simulink model "helipid"  (Simulink 7.7)
settings: Solver=ode45  StartTime=0.0  StopTime=2  RelTol=1e-3
values from neighbouring files (symbols this model uses):
  m = 97.85/2.20462262    (= 44.3840134417)    [heli_parameter.m]    (also in lin_thrust_countertorque.m; parameter.m)
undefined symbols (not defined in the file or in its folder): s
libraries: simulink x3, aerolib6dofsys x2, aerolibconvert2 x2, aerolibanim x1
settings Model: Creator=Administrator  LastModifiedBy=Li

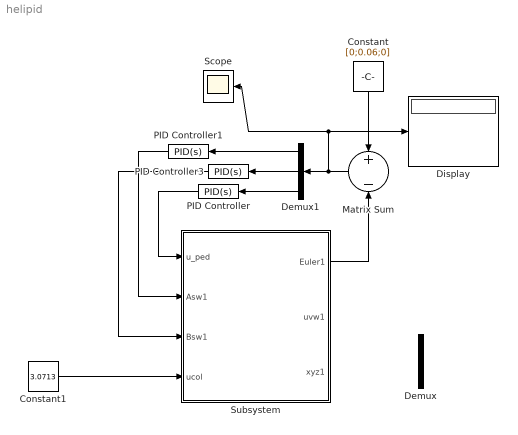
== system helipid ==
  Constant : Constant  Value=[0;0.06;0]
  Constant1 : Constant  Value=3.0713
  Demux : Demux  Outputs=3
  Demux1 : Demux  Outputs=3
  Display : Display
  Matrix Sum : Sum  Inputs=+-
  PID Controller : simulink/Continuous/PID Controller  SystemSampleTime=-1  Controller=PID  TimeDomain=Continuous-time  SampleTime=1  IntegratorMethod=Forward Euler  FilterMethod=Forward Euler  Form=Parallel  P=1  I=1  D=0  N=100  InitialConditionSource=internal  InitialConditionForIntegrator=0  InitialConditionForFilter=0  ExternalReset=none  LimitOutput=off  UpperSaturationLimit=inf  LowerSaturationLimit=-inf  LinearizeAsGain=off  AntiWindupMode=none  Kb=1  TrackingMode=off  Kt=1  PParamMin=[]  PParamMax=[]  IParamMin=[]  IParamMax=[]  DParamMin=[]  DParamMax=[]  NParamMin=[]  NParamMax=[]  KbParamMin=[]  KbParamMax=[]  KtParamMin=[]  KtParamMax=[]  POutMin=[]  POutMax=[]  IOutMin=[]  IOutMax=[]  DOutMin=[]  DOutMax=[]  NOutMin=[]  NOutMax=[]  KbOutMin=[]  KbOutMax=[]  KtOutMin=[]  KtOutMax=[]  IntegratorOutMin=[]  IntegratorOutMax=[]  FilterOutMin=[]  FilterOutMax=[]  SumOutMin=[]  SumOutMax=[]  SumI1OutMin=[]  SumI1OutMax=[]  SumI2OutMin=[]  SumI2OutMax=[]  SumI3OutMin=[]  SumI3OutMax=[]  SumDOutMin=[]  SumDOutMax=[]  SaturationOutMin=[]  SaturationOutMax=[]  IntegratorContinuousStateAttributes=''  IntegratorStateMustResolveToSignalObject=off  IntegratorRTWStateStorageClass=Auto  FilterContinuousStateAttributes=''  FilterStateMustResolveToSignalObject=off  FilterRTWStateStorageClass=Auto
  PID Controller1 : simulink/Continuous/PID Controller  SystemSampleTime=-1  Controller=PID  TimeDomain=Continuous-time  SampleTime=1  IntegratorMethod=Forward Euler  FilterMethod=Forward Euler  Form=Parallel  P=2  I=1  D=0.2  N=100  InitialConditionSource=internal  InitialConditionForIntegrator=0  InitialConditionForFilter=0  ExternalReset=none  LimitOutput=off  UpperSaturationLimit=inf  LowerSaturationLimit=-inf  LinearizeAsGain=off  AntiWindupMode=none  Kb=1  TrackingMode=off  Kt=1  PParamMin=[]  PParamMax=[]  IParamMin=[]  IParamMax=[]  DParamMin=[]  DParamMax=[]  NParamMin=[]  NParamMax=[]  KbParamMin=[]  KbParamMax=[]  KtParamMin=[]  KtParamMax=[]  POutMin=[]  POutMax=[]  IOutMin=[]  IOutMax=[]  DOutMin=[]  DOutMax=[]  NOutMin=[]  NOutMax=[]  KbOutMin=[]  KbOutMax=[]  KtOutMin=[]  KtOutMax=[]  IntegratorOutMin=[]  IntegratorOutMax=[]  FilterOutMin=[]  FilterOutMax=[]  SumOutMin=[]  SumOutMax=[]  SumI1OutMin=[]  SumI1OutMax=[]  SumI2OutMin=[]  SumI2OutMax=[]  SumI3OutMin=[]  SumI3OutMax=[]  SumDOutMin=[]  SumDOutMax=[]  SaturationOutMin=[]  SaturationOutMax=[]  IntegratorContinuousStateAttributes=''  IntegratorStateMustResolveToSignalObject=off  IntegratorRTWStateStorageClass=Auto  FilterContinuousStateAttributes=''  FilterStateMustResolveToSignalObject=off  FilterRTWStateStorageClass=Auto
  PID Controller3 : simulink/Continuous/PID Controller  SystemSampleTime=-1  Controller=PID  TimeDomain=Continuous-time  SampleTime=1  IntegratorMethod=Forward Euler  FilterMethod=Forward Euler  Form=Parallel  P=1.25  I=0.5  D=0.0474823432420019  N=10  InitialConditionSource=internal  InitialConditionForIntegrator=0  InitialConditionForFilter=0  ExternalReset=none  LimitOutput=off  UpperSaturationLimit=inf  LowerSaturationLimit=-inf  LinearizeAsGain=off  AntiWindupMode=none  Kb=1  TrackingMode=off  Kt=1  PParamMin=[]  PParamMax=[]  IParamMin=[]  IParamMax=[]  DParamMin=[]  DParamMax=[]  NParamMin=[]  NParamMax=[]  KbParamMin=[]  KbParamMax=[]  KtParamMin=[]  KtParamMax=[]  POutMin=[]  POutMax=[]  IOutMin=[]  IOutMax=[]  DOutMin=[]  DOutMax=[]  NOutMin=[]  NOutMax=[]  KbOutMin=[]  KbOutMax=[]  KtOutMin=[]  KtOutMax=[]  IntegratorOutMin=[]  IntegratorOutMax=[]  FilterOutMin=[]  FilterOutMax=[]  SumOutMin=[]  SumOutMax=[]  SumI1OutMin=[]  SumI1OutMax=[]  SumI2OutMin=[]  SumI2OutMax=[]  SumI3OutMin=[]  SumI3OutMax=[]  SumDOutMin=[]  SumDOutMax=[]  SaturationOutMin=[]  SaturationOutMax=[]  IntegratorContinuousStateAttributes=''  IntegratorStateMustResolveToSignalObject=off  IntegratorRTWStateStorageClass=Auto  FilterContinuousStateAttributes=''  FilterStateMustResolveToSignalObject=off  FilterRTWStateStorageClass=Auto
  Scope : Scope
      settings: SaveName=ScopeData13
  Subsystem : Subsystem
  wires:
  Constant/1 -> Matrix Sum/1
  Subsystem/1(Euler1) -> Matrix Sum/2
  Matrix Sum/1 -> Demux1/1, Display/1, Scope/1
  Demux1/3 -> PID Controller/1
  PID Controller/1 -> Subsystem/1(u_ped)
  Demux1/1 -> PID Controller1/1
  PID Controller1/1 -> Subsystem/2(Asw1)
  Demux1/2 -> PID Controller3/1
  PID Controller3/1 -> Subsystem/3(Bsw1)
  Constant1/1 -> Subsystem/4(ucol)

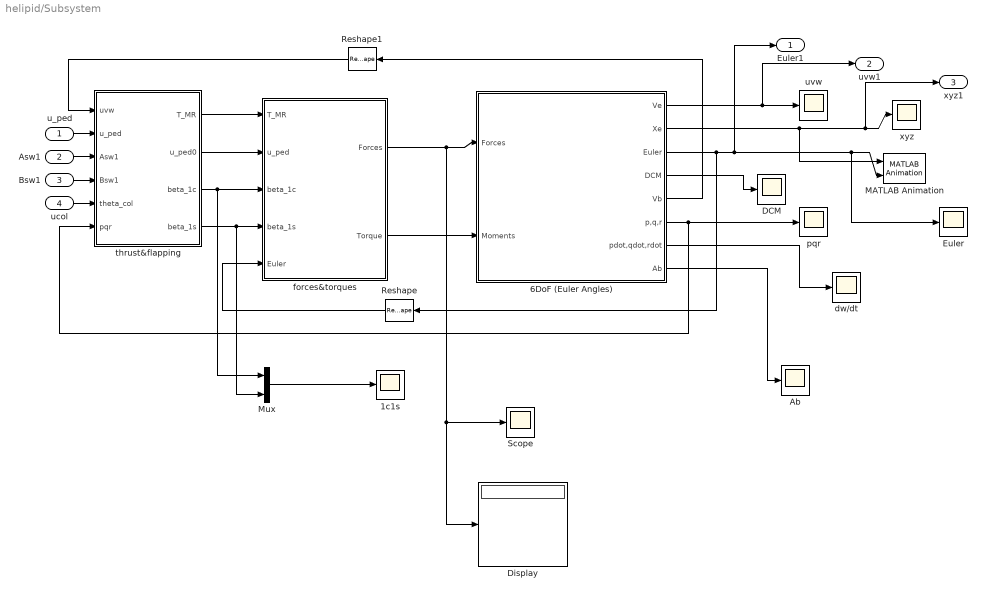
== system helipid/Subsystem ==
  u_ped : Inport
  Asw1 : Inport  Port=2
  Bsw1 : Inport  Port=3
  ucol : Inport  Port=4
  1c1s : Scope
      settings: YMin=1.5e-007  YMax=6.75e-007
  6DoF (Euler Angles) : Subsystem  AncestorBlock=aerolib6dof2/6DoF (Euler Angles)  mask(6DoF EoM (Body Axis)){units=Metric (MKS), mtype=Fixed, rep=Euler Angles, xme_0=[0;0;0], Vm_0=[0;0;0], eul_0=[0;0;0], pm_0=[0;0;0], mass_0=44.38401344172002, mass_e=0.5, mass_f=2.0, inertia=[1.4667965 0 0;0 4.5766695 0;0 0 4.407], inertia_e=eye(3), inertia_f=2*eye(3), k_quat=1.0}
      mask prompts: mtype "Mass type:"; rep "Representation:"; xme_0 "Initial position in inertial axes [Xe,Ye,Ze]:"; Vm_0 "Initial velocity in body axes [U,v,w]:"; eul_0 "Initial Euler orientation [roll, pitch, yaw]:"; pm_0 "Initial body rotation rates [p,q,r]:"; mass_0 "Initial mass:"; mass_e "Empty mass:"; mass_f "Full mass:"; inertia_e "Empty inertia matrix:"; inertia_f "Full inertia matrix:"; k_quat "Gain for quaternion normalization:"
      mask help: Integrate the six-degrees-of-freedom equations of motion in body axis.
      mask init:
      | [x y xp yp highstr lowstr maxy miny]=aeroimage('sixdofbody',gcbh);
      | ports=aeroicon('aeroblk6dofbody','icon');
      mask Help: eval('asbhelp(''sixdof_euler_angles'')');
      mask StyleString: popup(Metric (MKS)|English (Velocity in ft/s)|English (Velocity in kts)),popup(Fixed|Simple Variable|Custom Variable),popup(Euler Angles|Quaternion),edit,edit,edit,edit,edit,edit,edit,edit,edit,edit,edit
      mask CallbackString: |aeroicon('aeroblk6dofbody');|aeroicon('aeroblk6dofbody');|||||||||||
      mask Display:
      | port_label(ports(1).type,ports(1).port,ports(1).txt,'texmode','on');
      | port_label(ports(2).type,ports(2).port,ports(2).txt,'texmode','on');
      | port_label(ports(3).type,ports(3).port,ports(3).txt,'texmode','on');
      | port_label(ports(4).type,ports(4).port,ports(4).txt,'texmode','on');
      | port_label(ports(5).type,ports(5).port,ports(5).txt,'texmode','on');
      | port_label(ports(6).type,ports(6).port,ports(6).txt,'texmode','on');
      | port_label(ports(7).type,ports(7).port,ports(7).txt,'texmode','on');
      | port_label(ports(8).type,ports(8).port,ports(8).txt,'texmode','on');
      | port_label(ports(9).type,ports(9).port,ports(9).txt,'texmode','on');
      | port_label(ports(10).type,ports(10).port,ports(10).txt,'texmode','on');
      | port_label(ports(11).type,ports(11).port,ports(11).txt,'texmode','on');
      | port_label(ports(12).type,ports(12).port,ports(12).txt,'texmode','on');
      | port_label(ports(13).type,ports(13).port,ports(13).txt,'texmode','on');
      | port_label(ports(14).type,ports(14).port,ports(14).txt,'texmode','on');
      | port_label(ports(15).type,ports(15).port,ports(15).txt,'texmode','on');
      | text(0.5,maxy+0.065,highstr{:},'horizontalAlignment','center')
      | text(0.5,miny-0.05,lowstr{:},'horizontalAlignment','center')
      | plot(x,y);
      | patch(xp, yp);
  Ab : Scope
      settings: YMin=-2.5  YMax=0  SaveName=ScopeData12
  DCM : Scope
      settings: YMin=-2.5  YMax=0  SaveName=ScopeData11
  Display : Display
  Euler : Scope
      settings: YMin=-2.5  YMax=0
  MATLAB Animation : aerolibanim/MATLAB Animation  Vehicles=1  Geometries='astredwedge.mat'  BoundingBoxCoordinates=[-50,50,-50,50,-50,50]  CameraOffset=[-150,0,0]  CameraViewAngle=3  SampleTime=0.1  FigurePosition=[697,108,638,514]
  Mux : Mux  Inputs=2
  Reshape : Reshape  OutputDimensionality=Column vector (2-D)
  Reshape1 : Reshape  OutputDimensionality=Column vector (2-D)
  Scope : Scope
      settings: YMin=-2.5  YMax=0  SaveName=ScopeData2
  dw/dt : Scope
      settings: YMin=-2.5  YMax=0  SaveName=ScopeData3
  forces&torques : Subsystem  mask{mass0=44.384, AQ=0.00036, BQ=0.01, lm=0, ym=0, hm=0.2, Lt=1.2, Ht=0}
  pqr : Scope
      settings: YMin=-2.5  YMax=0  SaveName=ScopeData5
  thrust&flapping : Subsystem  mask{Ksw=0.2, Kcr=0.8, T_old=10, vi0=1, theta_twist=4.864e-4, theta_0=0.07}
  uvw : Scope
      settings: YMin=-2.5  YMax=0  SaveName=ScopeData6
  xyz : Scope
      settings: YMin=-2.5  YMax=0  SaveName=ScopeData7
  Euler1 : Outport
  uvw1 : Outport  Port=2
  xyz1 : Outport  Port=3
  wires:
  forces&torques/1(Forces) -> 6DoF (Euler Angles)/1(Forces), Scope/1, Display/1
  6DoF (Euler Angles)/6(p,q,r) -> thrust&flapping/6(pqr), pqr/1
  6DoF (Euler Angles)/3(Euler) -> Reshape/1, MATLAB Animation/2, Euler/1, Euler1/1
  thrust&flapping/1(T_MR) -> forces&torques/1(T_MR)
  thrust&flapping/2(u_ped0) -> forces&torques/2(u_ped)
  Reshape/1 -> forces&torques/5(Euler)
  6DoF (Euler Angles)/5(Vb) -> Reshape1/1
  Reshape1/1 -> thrust&flapping/1(uvw)
  thrust&flapping/3(beta_1c) -> forces&torques/3(beta_1c), Mux/1
  thrust&flapping/4(beta_1s) -> forces&torques/4(beta_1s), Mux/2
  forces&torques/2(Torque) -> 6DoF (Euler Angles)/2(Moments)
  Mux/1 -> 1c1s/1
  6DoF (Euler Angles)/1(Ve) -> uvw/1, uvw1/1
  6DoF (Euler Angles)/2(Xe) -> MATLAB Animation/1, xyz/1, xyz1/1
  6DoF (Euler Angles)/7(pdot,qdot,rdot) -> dw/dt/1
  6DoF (Euler Angles)/4(DCM) -> DCM/1
  u_ped/1 -> thrust&flapping/2(u_ped)
  Asw1/1 -> thrust&flapping/3(Asw1)
  Bsw1/1 -> thrust&flapping/4(Bsw1)
  ucol/1 -> thrust&flapping/5(theta_col)
  6DoF (Euler Angles)/8(Ab) -> Ab/1

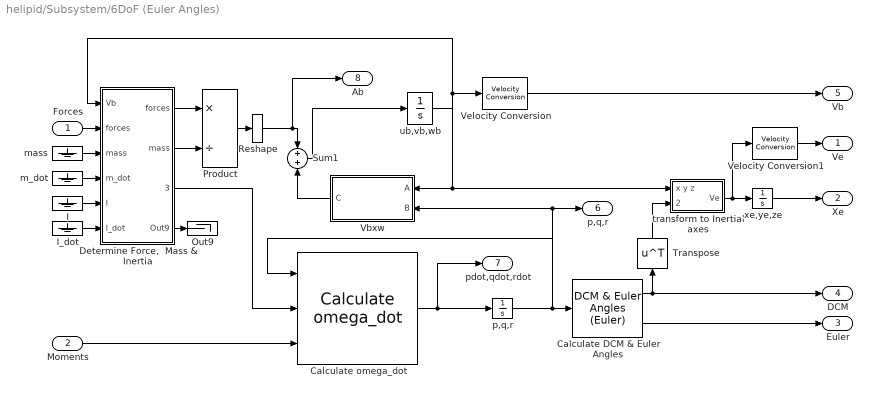
== system helipid/Subsystem/6DoF (Euler Angles) ==
  Forces : Inport
  Moments : Inport  Port=2
  Calculate DCM & Euler Angles : aerolib6dofsys/DCM & Euler Angles (Euler)  SystemSampleTime=-1
  Calculate omega_dot : aerolib6dofsys/Calculate omega_dot  SystemSampleTime=-1
  "Determine Force,  Mass & Inertia" : Subsystem  AncestorBlock=aerolib6dofsys/Mass & Inertia (fixed)
      mask Type: Mass & Inertia (fixed)
  I : Ground
  I_dot : Ground
  Out9 : Terminator
  Product : Product  Inputs=*/  SaturateOnIntegerOverflow=on  OutDataTypeStr=Inherit: Same as first input
  Reshape : Reshape  OutputDimensionality=Column vector (2-D)
  Sum1 : Sum  SaturateOnIntegerOverflow=on  InputSameDT=on  OutDataTypeStr=Inherit: Same as first input
  Transpose : Math  Operator=transpose  SaturateOnIntegerOverflow=on
  Vbxw : Subsystem  AncestorBlock=aerolibutil/3x3 Cross Product  mask(CrossProduct){}
      mask help: Calculate the cross product of two 3-by-1 vectors.
      mask init:
      | aeroicon('aeroblk');
      mask Help: eval('asbhelp(''threebythree_cross_product'')');
      mask Display:
      | text(.5,.5,'Cross\nProduct\nC = AxB', ...
      | 	'HorizontalAlignment','Center',...
      | 	'VerticalAlignment','middle')
  Velocity Conversion : aerolibconvert2/Velocity Conversion  SystemSampleTime=-1  IU=m/s  OU=m/s
  Velocity Conversion1 : aerolibconvert2/Velocity Conversion  SystemSampleTime=-1  IU=m/s  OU=m/s
  m_dot : Ground
  mass : Ground
  "p,q,r " : Integrator  InitialCondition=pm_0
  "transform to Inertial axes " : Subsystem
      mask Type: Vector Transformation
      mask Display: disp('L_EB')
  ub,vb,wb : Integrator  InitialCondition=convvel(Vm_0,'m/s','m/s')
  xe,ye,ze : Integrator  InitialCondition=xme_0
  Ve : Outport
  Xe : Outport  Port=2
  Euler : Outport  Port=3
  DCM : Outport  Port=4
  Vb : Outport  Port=5
  p,q,r : Outport  Port=6
  pdot,qdot,rdot : Outport  Port=7
  Ab : Outport  Port=8
  wires:
  "Determine Force,  Mass & Inertia"/1("forces ") -> Product/1
  I_dot/1 -> "Determine Force,  Mass & Inertia"/6(I_dot)
  I/1 -> "Determine Force,  Mass & Inertia"/5(I)
  Calculate omega_dot/1 -> "p,q,r "/1, pdot,qdot,rdot/1
  "Determine Force,  Mass & Inertia"/4(Out9) -> Out9/1
  m_dot/1 -> "Determine Force,  Mass & Inertia"/4(m_dot)
  "Determine Force,  Mass & Inertia"/2(mass) -> Product/2
  mass/1 -> "Determine Force,  Mass & Inertia"/3("mass ")
  Transpose/1 -> "transform to Inertial axes "/2(transform coefficients)
  Calculate DCM & Euler Angles/1 -> Transpose/1, DCM/1
  Forces/1 -> "Determine Force,  Mass & Inertia"/2(forces)
  Moments/1 -> Calculate omega_dot/3
  "p,q,r "/1 -> Calculate omega_dot/1, Calculate DCM & Euler Angles/1, Vbxw/2(B), p,q,r/1
  "transform to Inertial axes "/1(Ve) -> xe,ye,ze/1, Velocity Conversion1/1
  xe,ye,ze/1 -> Xe/1
  Sum1/1 -> ub,vb,wb/1
  ub,vb,wb/1 -> "Determine Force,  Mass & Inertia"/1(Vb), Vbxw/1(A), "transform to Inertial axes "/1(x y z), Velocity Conversion/1
  Vbxw/1(C) -> Sum1/2
  Calculate DCM & Euler Angles/2 -> Euler/1
  "Determine Force,  Mass & Inertia"/3("inertia, 0") -> Calculate omega_dot/2
  Velocity Conversion/1 -> Vb/1
  Velocity Conversion1/1 -> Ve/1
  Product/1 -> Reshape/1
  Reshape/1 -> Sum1/1, Ab/1

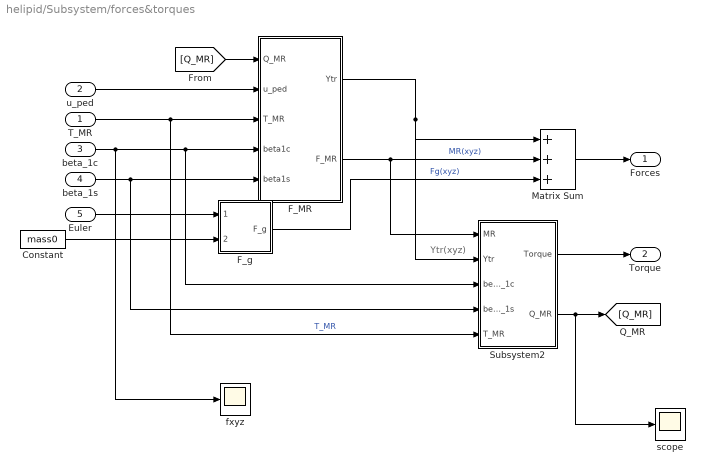
== system helipid/Subsystem/forces&torques ==
  note: Ytr(xyz)
  T_MR : Inport
  u_ped : Inport  Port=2
  beta_1c : Inport  Port=3
  beta_1s : Inport  Port=4
  Euler : Inport  Port=5
  Constant : Constant  Value=mass0
  F_MR : Subsystem
  F_g : Subsystem
  Matrix Sum : Sum  Inputs=+++  CollapseMode=Specified dimension  CollapseDim=3
  Subsystem2 : Subsystem
  fxyz : Scope
      settings: YMin=-37.5  YMax=10  SaveName=ScopeData9
  scope : Scope
      settings: YMin=-37.5  YMax=10  SaveName=ScopeData14
  Forces : Outport
  Torque : Outport  Port=2
  wires:
  F_MR/1(Ytr) -> Subsystem2/2(Ytr), Matrix Sum/1
  u_ped/1 -> F_MR/2(u_ped)
  Matrix Sum/1 -> Forces/1
  Subsystem2/1(Torque) -> Torque/1
  Constant/1 -> F_g/2(mass)
  F_g/1(F_g) -> Matrix Sum/3  "Fg(xyz)"
  Euler/1 -> F_g/1(Euler)
  T_MR/1 -> Subsystem2/5(T_MR), F_MR/3(T_MR)  "T_MR"
  Subsystem2/2(Q_MR) -> [Q_MR], scope/1
  [Q_MR] -> F_MR/1(Q_MR)
  beta_1c/1 -> F_MR/4(beta1c), Subsystem2/3(beta_1c), fxyz/1
  beta_1s/1 -> F_MR/5(beta1s), Subsystem2/4(beta_1s)
  F_MR/2(F_MR) -> Subsystem2/1(MR), Matrix Sum/2  "MR(xyz)"

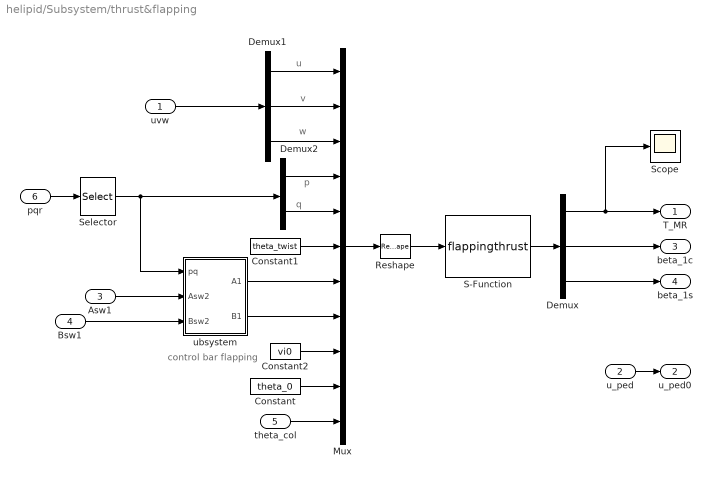
== system helipid/Subsystem/thrust&flapping ==
  note: p
  note: q
  note: u
  note: v
  note: w
  note: control bar flapping
  uvw : Inport
  u_ped : Inport  Port=2
  Asw1 : Inport  Port=3
  Bsw1 : Inport  Port=4
  theta_col : Inport  Port=5
  pqr : Inport  Port=6
  Constant : Constant  Value=theta_0
  Constant1 : Constant  Value=theta_twist
  Constant2 : Constant  Value=vi0
  Demux : Demux  Outputs=3
  Demux1 : Demux  Outputs=[1 1 1 ]
  Demux2 : Demux  Outputs=[1 1]
  Mux : Mux  Inputs=11
  Reshape : Reshape  OutputDimensionality=Column vector (2-D)
  S-Function : S-Function  RequirementInfo={} %GIDa_65d95cac_1915_47d0_9bf9_1f0f9807395a  FunctionName=flappingthrust  EnableBusSupport=off
  Scope : Scope
      settings: SaveName=ScopeData4
  Selector : Selector  InputPortWidth=3  IndexOptions=Index vector (dialog)  Indices=[1 2]  OutputSizes=1
  ubsystem : Subsystem
  T_MR : Outport
  u_ped0 : Outport  Port=2
  beta_1c : Outport  Port=3
  beta_1s : Outport  Port=4
  wires:
  u_ped/1 -> u_ped0/1
  S-Function/1 -> Demux/1
  Demux/1 -> T_MR/1, Scope/1
  Demux/2 -> beta_1c/1
  Demux1/1 -> Mux/1
  Demux1/2 -> Mux/2
  Demux1/3 -> Mux/3
  uvw/1 -> Demux1/1
  Demux2/1 -> Mux/4
  Demux2/2 -> Mux/5
  Constant2/1 -> Mux/9
  Demux/3 -> beta_1s/1
  Constant/1 -> Mux/10
  Mux/1 -> Reshape/1
  Reshape/1 -> S-Function/1
  Asw1/1 -> ubsystem/2(Asw2)
  Bsw1/1 -> ubsystem/3(Bsw2)
  ubsystem/1(A1) -> Mux/7
  ubsystem/2(B1) -> Mux/8
  theta_col/1 -> Mux/11
  Constant1/1 -> Mux/6
  pqr/1 -> Selector/1
  Selector/1 -> Demux2/1, ubsystem/1(pq)

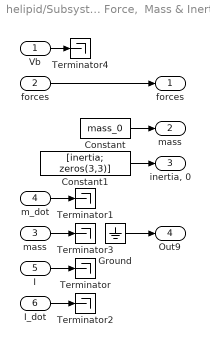
== system helipid/Subsystem/6DoF (Euler Angles)/Determine Force,  Mass & Inertia ==
  Vb : Inport
  forces : Inport  Port=2  PortDimensions=3
  "mass " : Inport  Port=3
  m_dot : Inport  Port=4  OutDataTypeStr=double
  I : Inport  Port=5  OutDataTypeStr=double
  I_dot : Inport  Port=6  OutDataTypeStr=double
  Constant : Constant  Value=mass_0  OutDataTypeStr=Inherit: Inherit via back propagation
  Constant1 : Constant  Value=[inertia; zeros(3,3)]  OutDataTypeStr=Inherit: Inherit via back propagation
  Ground : Ground
  Terminator{,1..4} (5 alike) : Terminator
  "forces " : Outport  PortDimensions=3
  mass : Outport  Port=2
  "inertia, 0" : Outport  Port=3
  Out9 : Outport  Port=4
  wires:
  Vb/1 -> Terminator4/1
  forces/1 -> "forces "/1
  "mass "/1 -> Terminator3/1
  I_dot/1 -> Terminator2/1
  m_dot/1 -> Terminator1/1
  I/1 -> Terminator/1
  Ground/1 -> Out9/1
  Constant1/1 -> "inertia, 0"/1
  Constant/1 -> mass/1

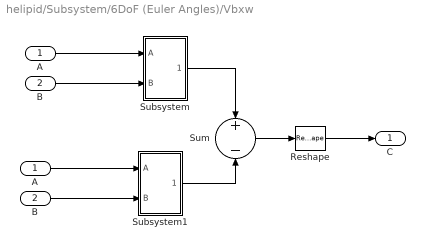
== system helipid/Subsystem/6DoF (Euler Angles)/Vbxw ==
  A : Inport  PortDimensions=3
  B : Inport  Port=2
  "A " : InportShadow  Port=1  PortDimensions=3
  "B " : InportShadow  Port=2
  Reshape : Reshape  OutputDimensionality=Column vector (2-D)
  Subsystem : Subsystem
  Subsystem1 : Subsystem
  Sum : Sum  Inputs=+|-  SaturateOnIntegerOverflow=on  InputSameDT=on  OutDataTypeStr=Inherit: Same as first input
  C : Outport
  wires:
  "B "/1 -> Subsystem1/2(B)
  "A "/1 -> Subsystem1/1(A)
  B/1 -> Subsystem/2(B)
  A/1 -> Subsystem/1(A)
  Subsystem/1(Out1) -> Sum/1
  Subsystem1/1(Out1) -> Sum/2
  Sum/1 -> Reshape/1
  Reshape/1 -> C/1

== system helipid/Subsystem/6DoF (Euler Angles)/transform to Inertial axes  ==
  x y z : Inport
  transform coefficients : Inport  Port=2
  Product : Product  Multiplication=Matrix(*)  SaturateOnIntegerOverflow=on  InputSameDT=on  OutDataTypeStr=Inherit: Same as first input
  Reshape1 : Reshape  OutputDimensionality=Column vector (2-D)
  Reshape2 : Reshape
  Ve : Outport
  wires:
  Reshape2/1 -> Ve/1
  Reshape1/1 -> Product/2
  x y z/1 -> Reshape1/1
  transform coefficients/1 -> Product/1
  Product/1 -> Reshape2/1

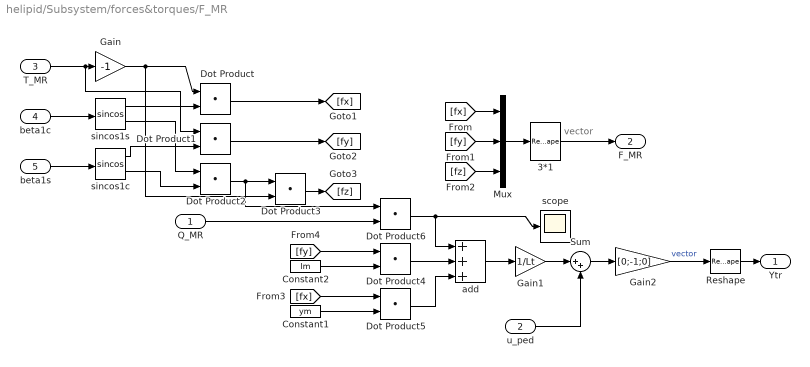
== system helipid/Subsystem/forces&torques/F_MR ==
  note: vector
  Q_MR : Inport
  u_ped : Inport  Port=2
  T_MR : Inport  Port=3
  beta1c : Inport  Port=4
  beta1s : Inport  Port=5
  3*1 : Reshape  OutputDimensionality=Column vector (2-D)
  Constant1 : Constant  Value=ym
  Constant2 : Constant  Value=lm
  Dot Product{,1..6} (7 alike) : DotProduct  InputSameDT=on  OutDataTypeStr=Inherit: Inherit via internal rule
  Gain : Gain  Gain=-1
  Gain1 : Gain  Gain=1/Lt
  Gain2 : Gain  Gain=[0;-1;0]
  Mux : Mux  Inputs=3
  Reshape : Reshape  OutputDimensionality=Column vector (2-D)
  Sum : Sum  Inputs=|++
  add : Sum  Inputs=+++
  scope : Scope
      settings: YMin=-37.5  YMax=10  SaveName=ScopeData15
  sincos1c : Trigonometry  Operator=sincos
  sincos1s : Trigonometry  Operator=sincos
  Ytr : Outport
  F_MR : Outport  Port=2
  wires:
  u_ped/1 -> Sum/2
  Gain1/1 -> Sum/1
  add/1 -> Gain1/1
  Q_MR/1 -> Dot Product6/2
  Constant1/1 -> Dot Product5/2
  Constant2/1 -> Dot Product4/2
  Mux/1 -> 3*1/1
  beta1s/1 -> sincos1c/1
  beta1c/1 -> sincos1s/1
  Dot Product2/1 -> Dot Product6/1, Dot Product3/1
  sincos1c/2 -> Dot Product2/2
  sincos1s/2 -> Dot Product2/1
  sincos1c/1 -> Dot Product1/2
  sincos1s/1 -> Dot Product/2
  Gain/1 -> Dot Product3/2, Dot Product/1
  Dot Product/1 -> [fx]
  Dot Product1/1 -> [fy]
  Dot Product3/1 -> [fz]
  [fx] -> Mux/1
  [fy] -> Mux/2
  [fz] -> Mux/3
  [fy] -> Dot Product4/1
  [fx] -> Dot Product5/1
  Dot Product6/1 -> add/1, scope/1
  Dot Product4/1 -> add/2
  Dot Product5/1 -> add/3
  Sum/1 -> Gain2/1
  Gain2/1 -> Reshape/1  "vector"
  Reshape/1 -> Ytr/1
  3*1/1 -> F_MR/1
  T_MR/1 -> Dot Product1/1, Gain/1

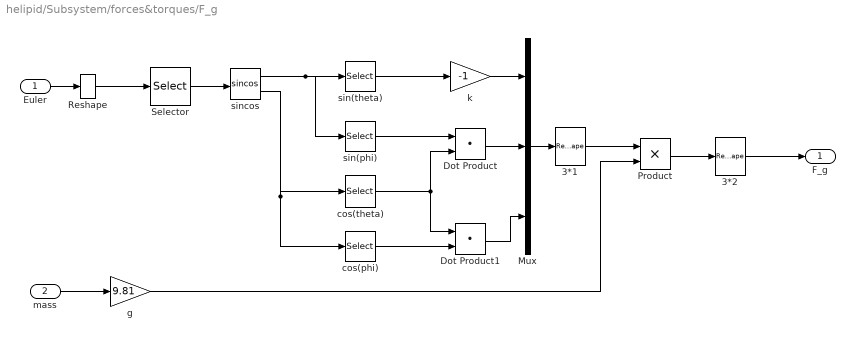
== system helipid/Subsystem/forces&torques/F_g ==
  Euler : Inport
  mass : Inport  Port=2  PortDimensions=1
  3*1 : Reshape  OutputDimensionality=Column vector (2-D)
  3*2 : Reshape  OutputDimensionality=Column vector (2-D)
  Dot Product : DotProduct  InputSameDT=on  OutDataTypeStr=Inherit: Inherit via internal rule
  Dot Product1 : DotProduct  InputSameDT=on  OutDataTypeStr=Inherit: Inherit via internal rule
  Mux : Mux  Inputs=3
  Product : Product  RndMeth=Zero
  Reshape : Reshape  OutputDimensionality=Column vector (2-D)
  Selector : Selector  InputPortWidth=3  IndexOptions=Index vector (dialog)  Indices=[1 2]  OutputSizes=1
  cos(phi) : Selector  InputPortWidth=2  IndexOptions=Index vector (dialog)  Indices=[1]  OutputSizes=1
  cos(theta) : Selector  InputPortWidth=2  IndexOptions=Index vector (dialog)  Indices=[2]  OutputSizes=1
  g : Gain  Gain=9.81
  k : Gain  Gain=-1
  sin(phi) : Selector  InputPortWidth=2  IndexOptions=Index vector (dialog)  Indices=[1]  OutputSizes=1
  sin(theta) : Selector  InputPortWidth=2  IndexOptions=Index vector (dialog)  Indices=[2]  OutputSizes=1
  sincos : Trigonometry  Operator=sincos
  F_g : Outport
  wires:
  cos(phi)/1 -> Dot Product1/2
  Reshape/1 -> Selector/1
  Euler/1 -> Reshape/1
  mass/1 -> g/1
  Dot Product1/1 -> Mux/3
  Dot Product/1 -> Mux/2
  cos(theta)/1 -> Dot Product1/1, Dot Product/2
  sin(phi)/1 -> Dot Product/1
  k/1 -> Mux/1
  sin(theta)/1 -> k/1
  sincos/2 -> cos(theta)/1, cos(phi)/1
  sincos/1 -> sin(theta)/1, sin(phi)/1
  Selector/1 -> sincos/1
  Mux/1 -> 3*1/1
  3*1/1 -> Product/1
  g/1 -> Product/2
  Product/1 -> 3*2/1
  3*2/1 -> F_g/1

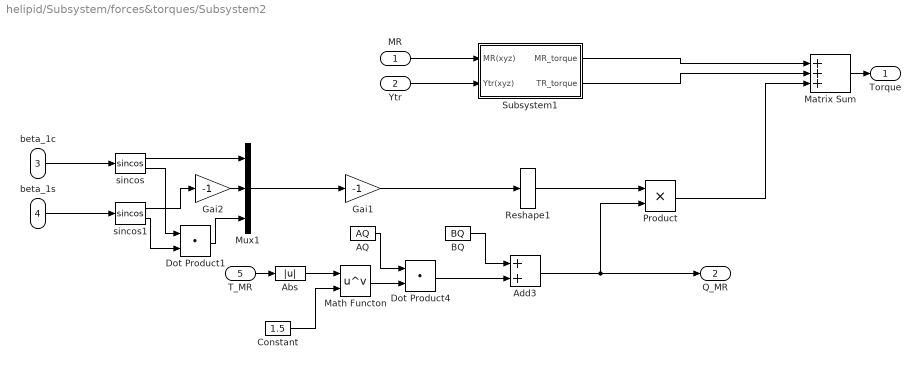
== system helipid/Subsystem/forces&torques/Subsystem2 ==
  MR : Inport  PortDimensions=3
  Ytr : Inport  Port=2  PortDimensions=3
  beta_1c : Inport  Port=3  PortDimensions=1
  beta_1s : Inport  Port=4  PortDimensions=1
  T_MR : Inport  Port=5
  AQ : Constant  Value=AQ
  Abs : Abs
  Add3 : Sum
  BQ : Constant  Value=BQ  VectorParams1D=off
  Constant : Constant  Value=1.5
  Dot Product1 : DotProduct  InputSameDT=on  OutDataTypeStr=Inherit: Inherit via internal rule
  Dot Product4 : DotProduct  InputSameDT=on  OutDataTypeStr=Inherit: Inherit via internal rule
  Gai1 : Gain  Gain=-1
  Gai2 : Gain  Gain=-1
  Math Functon : Math  Operator=pow  SaturateOnIntegerOverflow=on
  Matrix Sum : Sum  Inputs=+++  CollapseMode=Specified dimension  CollapseDim=3
  Mux1 : Mux  Inputs=3
  Product : Product  RndMeth=Zero
  Reshape1 : Reshape  OutputDimensionality=Column vector (2-D)
  Subsystem1 : Subsystem
  sincos : Trigonometry  Operator=sincos
  sincos1 : Trigonometry  Operator=sincos
  Torque : Outport
  Q_MR : Outport  Port=2
  wires:
  Matrix Sum/1 -> Torque/1
  beta_1s/1 -> sincos1/1
  beta_1c/1 -> sincos/1
  Ytr/1 -> Subsystem1/2(Ytr(xyz))
  MR/1 -> Subsystem1/1(MR(xyz))
  Subsystem1/2(TR_torque) -> Matrix Sum/2
  Subsystem1/1(MR_torque) -> Matrix Sum/1
  Dot Product1/1 -> Mux1/3
  sincos/2 -> Dot Product1/1
  sincos1/2 -> Dot Product1/2
  Gai2/1 -> Mux1/2
  sincos1/1 -> Gai2/1
  sincos/1 -> Mux1/1
  Dot Product4/1 -> Add3/2
  BQ/1 -> Add3/1
  AQ/1 -> Dot Product4/1
  Math Functon/1 -> Dot Product4/2
  Constant/1 -> Math Functon/2
  Product/1 -> Matrix Sum/3
  Reshape1/1 -> Product/1
  T_MR/1 -> Abs/1
  Abs/1 -> Math Functon/1
  Add3/1 -> Product/2, Q_MR/1
  Mux1/1 -> Gai1/1
  Gai1/1 -> Reshape1/1

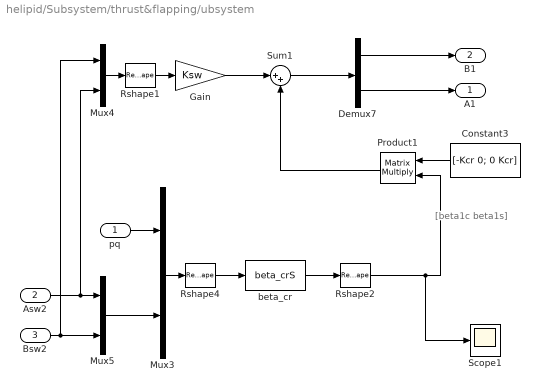
== system helipid/Subsystem/thrust&flapping/ubsystem ==
  note: [beta1c
      | beta1s]
  pq : Inport
  Asw2 : Inport  Port=2
  Bsw2 : Inport  Port=3
  Constant3 : Constant  Value=[-Kcr 0; 0 Kcr]
  Demux7 : Demux  Outputs=[1 1]
  Gain : Gain  Gain=Ksw
  Mux3 : Mux  Inputs=2
  Mux4 : Mux  Inputs=2
  Mux5 : Mux  Inputs=2
  Product1 : Product  Multiplication=Matrix(*)  RndMeth=Zero
  Rshape1 : Reshape  OutputDimensionality=Column vector (2-D)
  Rshape2 : Reshape  OutputDimensionality=Column vector (2-D)
  Rshape4 : Reshape  OutputDimensionality=Column vector (2-D)
  Scope1 : Scope
      settings: YMin=-1  YMax=2  SaveName=ScopeData8
  Sum1 : Sum  Inputs=|++
  beta_cr : S-Function  FunctionName=beta_crS  EnableBusSupport=off
  A1 : Outport
  B1 : Outport  Port=2
  wires:
  Rshape4/1 -> beta_cr/1
  Mux3/1 -> Rshape4/1
  Product1/1 -> Sum1/2
  Mux4/1 -> Rshape1/1
  Rshape1/1 -> Gain/1
  Sum1/1 -> Demux7/1
  Gain/1 -> Sum1/1
  Constant3/1 -> Product1/1
  Bsw2/1 -> Mux5/2, Mux4/1
  Asw2/1 -> Mux5/1, Mux4/2
  Demux7/1 -> B1/1
  Demux7/2 -> A1/1
  beta_cr/1 -> Rshape2/1
  Rshape2/1 -> Product1/2, Scope1/1
  Mux5/1 -> Mux3/2
  pq/1 -> Mux3/1

== system helipid/Subsystem/6DoF (Euler Angles)/Vbxw/Subsystem ==
  A : Inport
  B : Inport  Port=2
  Demux : Demux  Outputs=3
  Demux1 : Demux  Outputs=3
  Mux : Mux  Inputs=3
  i x j : Product  SaturateOnIntegerOverflow=on  InputSameDT=on  OutDataTypeStr=Inherit: Same as first input
  j x k : Product  SaturateOnIntegerOverflow=on  InputSameDT=on  OutDataTypeStr=Inherit: Same as first input
  k x i : Product  SaturateOnIntegerOverflow=on  InputSameDT=on  OutDataTypeStr=Inherit: Same as first input
  Out1 : Outport  PortDimensions=3
  wires:
  Demux1/3 -> j x k/2
  Demux/2 -> j x k/1
  Demux/3 -> k x i/1
  Demux1/1 -> k x i/2
  Demux1/2 -> i x j/2
  Demux/1 -> i x j/1
  i x j/1 -> Mux/3
  k x i/1 -> Mux/2
  j x k/1 -> Mux/1
  B/1 -> Demux1/1
  A/1 -> Demux/1
  Mux/1 -> Out1/1

== system helipid/Subsystem/6DoF (Euler Angles)/Vbxw/Subsystem1 ==
  A : Inport
  B : Inport  Port=2
  Demux : Demux  Outputs=3
  Demux1 : Demux  Outputs=3
  Mux : Mux  Inputs=3
  i x k : Product  SaturateOnIntegerOverflow=on  InputSameDT=on  OutDataTypeStr=Inherit: Same as first input
  j x i : Product  SaturateOnIntegerOverflow=on  InputSameDT=on  OutDataTypeStr=Inherit: Same as first input
  k x j : Product  SaturateOnIntegerOverflow=on  InputSameDT=on  OutDataTypeStr=Inherit: Same as first input
  Out1 : Outport  PortDimensions=3
  wires:
  j x i/1 -> Mux/3
  i x k/1 -> Mux/2
  k x j/1 -> Mux/1
  Mux/1 -> Out1/1
  Demux1/1 -> j x i/2
  Demux/2 -> j x i/1
  Demux1/3 -> i x k/2
  Demux/1 -> i x k/1
  Demux1/2 -> k x j/2
  Demux/3 -> k x j/1
  B/1 -> Demux1/1
  A/1 -> Demux/1

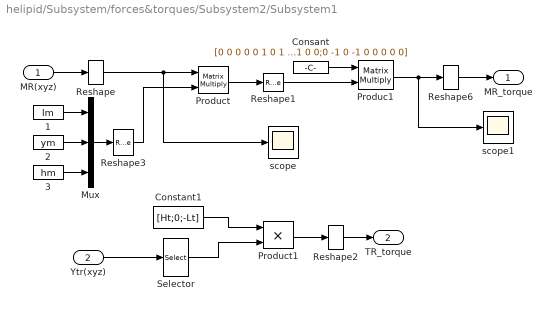
== system helipid/Subsystem/forces&torques/Subsystem2/Subsystem1 ==
  MR(xyz) : Inport
  Ytr(xyz) : Inport  Port=2
  1 : Constant  Value=lm
  2 : Constant  Value=ym
  3 : Constant  Value=hm
  Consant : Constant  Value=[0 0 0 0 0 1 0 1 0;0 0 1 0 0 0 -1 0 0;0 -1 0 -1 0 0 0 0 0]
  Constant1 : Constant  Value=[Ht;0;-Lt]
  Mux : Mux  Inputs=3
  Produc1 : Product  Multiplication=Matrix(*)  RndMeth=Zero
  Product : Product  Multiplication=Matrix(*)  RndMeth=Zero
  Product1 : Product  RndMeth=Zero
  Reshape{,1..2,6} (4 alike) : Reshape  OutputDimensionality=Column vector (2-D)
  Reshape3 : Reshape  OutputDimensionality=Row vector (2-D)
  Selector : Selector  InputPortWidth=3  IndexOptions=Index vector (dialog)  Indices=[2]  OutputSizes=1
  scope : Scope
      settings: YMin=-37.5  YMax=10  SaveName=ScopeData10
  scope1 : Scope
      settings: YMin=-37.5  YMax=10  SaveName=ScopeData16
  MR_torque : Outport
  TR_torque : Outport  Port=2
  wires:
  Reshape6/1 -> MR_torque/1
  Produc1/1 -> Reshape6/1, scope1/1
  Consant/1 -> Produc1/1
  Reshape1/1 -> Produc1/2
  Ytr(xyz)/1 -> Selector/1
  Product/1 -> Reshape1/1
  Reshape3/1 -> Product/2
  Reshape/1 -> Product/1, scope/1
  Mux/1 -> Reshape3/1
  MR(xyz)/1 -> Reshape/1
  3/1 -> Mux/3
  2/1 -> Mux/2
  1/1 -> Mux/1
  Product1/1 -> Reshape2/1
  Reshape2/1 -> TR_torque/1
  Constant1/1 -> Product1/1
  Selector/1 -> Product1/2
